simulink model "room_heating_2004"  (R2017b)
settings: Solver=VariableStepAuto  StartTime=0.0  StopTime=600  RelTol=1e-3
StopFcn:
  | time=T_Raum.time;
  | time=time/24+737902;
  | time=datetime(time,'ConvertFrom','datenum');
  | TT=timetable(time,T_Raum.data,T_tank.data,'VariableNames',{'T_room','T_tank'});
  | TT=timetable2table(TT);
  | writetable(TT,'test01.csv');
  | TT2=timetable(time,T_aussen.data,'VariableNames',{'T_outside'});
  | TT2=timetable2table(TT2);
  | writetable(TT2,'test02.csv');
model workspace (MAT data in the model file):
  I_Heizelement = 1800000
  R_Oberflaeche = 1.035e-06
  R_los = 0.00036552
  Ts = 0.777928481401
  c_Luft = 1005
  c_Wasser = 4184
  ks = 0.997176412817
  m_Kessel = 150
  m_Raumluft = 750
libraries: simulink x1
settings Model: Creator=y03li  LastModifiedBy=y03li

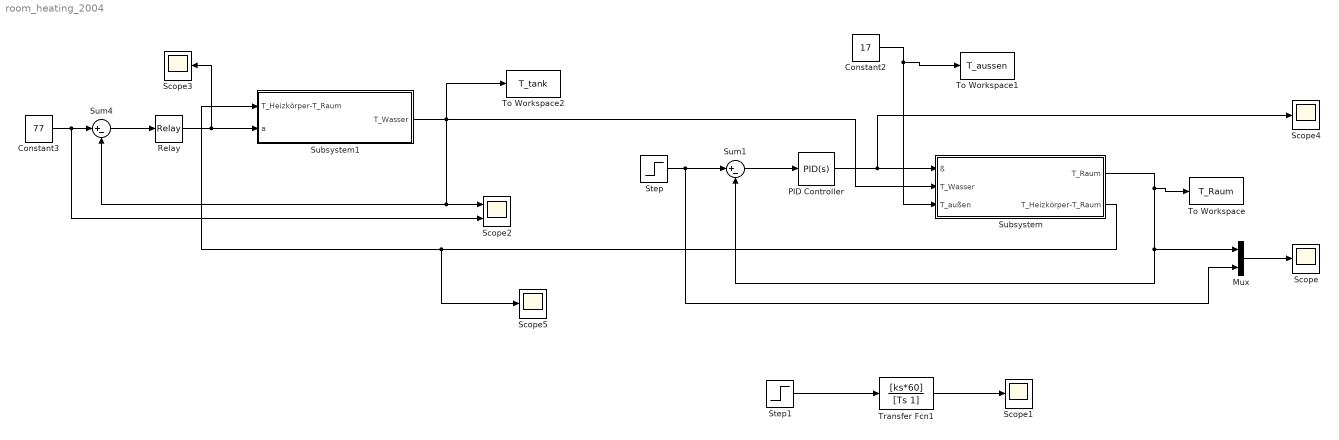
== system room_heating_2004 ==
  Constant2 : Constant  Value=17
  Constant3 : Constant  Value=77
  Mux : Mux  Inputs=2
  PID Controller : simulink/Continuous/PID Controller  Controller=PID  TimeDomain=Continuous-time  SampleTime=-1  IntegratorMethod=Forward Euler  FilterMethod=Forward Euler  Form=Parallel  UseFilter=on  ControllerParametersSource=internal  P=0.5/(ks*60)  I=0.5/(ks*60*0.8*Ts)  D=0  N=100  InitialConditionSource=internal  InitialConditionForIntegrator=0  InitialConditionForFilter=0  ExternalReset=none  LimitOutput=off  UpperSaturationLimit=1  LowerSaturationLimit=0  LinearizeAsGain=on  AntiWindupMode=none  Kb=1  TrackingMode=off  Kt=1  PParamMin=[]  PParamMax=[]  IParamMin=[]  IParamMax=[]  DParamMin=[]  DParamMax=[]  NParamMin=[]  NParamMax=[]  KbParamMin=[]  KbParamMax=[]  KtParamMin=[]  KtParamMax=[]  POutMin=[]  POutMax=[]  IOutMin=[]  IOutMax=[]  DOutMin=[]  DOutMax=[]  NOutMin=[]  NOutMax=[]  KbOutMin=[]  KbOutMax=[]  KtOutMin=[]  KtOutMax=[]  IntegratorOutMin=[]  IntegratorOutMax=[]  FilterOutMin=[]  FilterOutMax=[]  SumOutMin=[]  SumOutMax=[]  SumI1OutMin=[]  SumI1OutMax=[]  SumI2OutMin=[]  SumI2OutMax=[]  SumI3OutMin=[]  SumI3OutMax=[]  SumDOutMin=[]  SumDOutMax=[]  SaturationOutMin=[]  SaturationOutMax=[]  IntegratorContinuousStateAttributes=''  IntegratorStateMustResolveToSignalObject=off  IntegratorRTWStateStorageClass=Auto  FilterContinuousStateAttributes=''  FilterStateMustResolveToSignalObject=off  FilterRTWStateStorageClass=Auto  DifferentiatorICPrevScaledInput=0  DifferentiatorOutMin=[]  DifferentiatorOutMax=[]  InitialConditionSetting=State (most efficient)  FilterDiffOutCoefMin=[]  FilterDiffOutCoefMax=[]  SumDenOutMin=[]  SumDenOutMax=[]  SumNumOutMin=[]  SumNumOutMax=[]  ReciprocalOutMin=[]  ReciprocalOutMax=[]  DivideOutMin=[]  DivideOutMax=[]  TunerSelectOption=Transfer Function Based (PID Tuner App)
  Relay : Relay  OnSwitchValue=0.5  OffSwitchValue=-0.5
  Scope{,1,3..5} (5 alike) : Scope
  Scope2 : Scope  NumInputPorts=2
  Step : Step  Time=0  Before=20  After=20  SampleTime=0
  Step1 : Step  Time=0  SampleTime=0
  Subsystem : Subsystem
  Subsystem1 : Subsystem
  Sum1 : Sum  Inputs=|+-
  Sum4 : Sum  Inputs=|+-
  To Workspace : ToWorkspace  VariableName=T_Raum  SaveFormat=Timeseries  SampleTime=-1
      settings: Save2DSignal=2-D array (concatenate along first dimension)
  To Workspace1 : ToWorkspace  VariableName=T_aussen  SaveFormat=Timeseries  SampleTime=-1
      settings: Save2DSignal=2-D array (concatenate along first dimension)
  To Workspace2 : ToWorkspace  VariableName=T_tank  SaveFormat=Timeseries  SampleTime=-1
      settings: Save2DSignal=2-D array (concatenate along first dimension)
  Transfer Fcn1 : TransferFcn  Numerator=[ks*60]  Denominator=[Ts 1]
  wires:
  Sum1/1 -> PID Controller/1
  Step/1 -> Mux/2, Sum1/1
  Mux/1 -> Scope/1
  Transfer Fcn1/1 -> Scope1/1
  Step1/1 -> Transfer Fcn1/1
  Subsystem/1(T_Raum) -> To Workspace/1, Mux/1, Sum1/2
  PID Controller/1 -> Scope4/1, Subsystem/1(ß)
  Constant2/1 -> To Workspace1/1, Subsystem/3(T_außen)
  Relay/1 -> Subsystem1/2(a), Scope3/1
  Constant3/1 -> Scope2/2, Sum4/1
  Sum4/1 -> Relay/1
  Subsystem/2(T_Heizkörper-T_Raum) -> Scope5/1, Subsystem1/1(T_Heizkörper-T_Raum)
  Subsystem1/1(T_Wasser) -> Subsystem/2(T_Wasser), To Workspace2/1, Scope2/1, Sum4/2

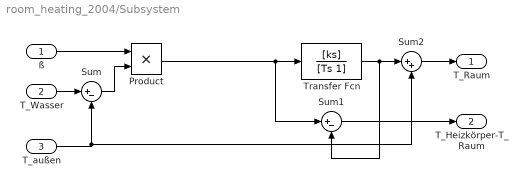
== system room_heating_2004/Subsystem ==
  ß : Inport
  T_Wasser : Inport  Port=2
  T_außen : Inport  Port=3
  Product : Product
  Sum : Sum  Inputs=|+-
  Sum1 : Sum  Inputs=|+-
  Sum2 : Sum  Inputs=|++
  Transfer Fcn : TransferFcn  Numerator=[ks]  Denominator=[Ts 1]
  T_Raum : Outport
  T_Heizkörper-T_Raum : Outport  Port=2
  wires:
  ß/1 -> Product/1
  Transfer Fcn/1 -> Sum1/2, Sum2/1
  Sum2/1 -> T_Raum/1
  Sum/1 -> Product/2
  Product/1 -> Sum1/1, Transfer Fcn/1
  T_Wasser/1 -> Sum/1
  T_außen/1 -> Sum2/2, Sum/2
  Sum1/1 -> T_Heizkörper-T_Raum/1

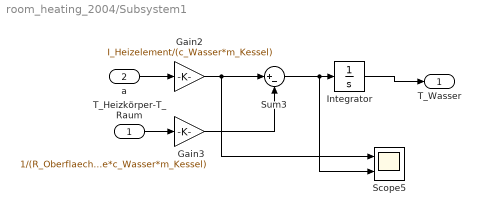
== system room_heating_2004/Subsystem1 ==
  T_Heizkörper-T_Raum : Inport
  a : Inport  Port=2
  Gain2 : Gain  Gain=I_Heizelement/(c_Wasser*m_Kessel)
  Gain3 : Gain  Gain=1/(R_Oberflaeche*c_Wasser*m_Kessel)
  Integrator : Integrator  InitialCondition=20
  Scope5 : Scope  NumInputPorts=2
  Sum3 : Sum  Inputs=|+-
  T_Wasser : Outport
  wires:
  Gain2/1 -> Scope5/1, Sum3/1
  a/1 -> Gain2/1
  Integrator/1 -> T_Wasser/1
  Gain3/1 -> Sum3/2
  Sum3/1 -> Scope5/2, Integrator/1
  T_Heizkörper-T_Raum/1 -> Gain3/1
